simulink model "A2_TwoDOF_PID_task_space"  (R2014a)
settings: Solver=ode23t  StartTime=0.0  StopTime=10  FixedStep=1e-5  RelTol=1e-3
undefined symbols (not defined in the file): ADAMS_cwd, ADAMS_exec, ADAMS_host, ADAMS_init, ADAMS_inputs, ADAMS_outputs, ADAMS_prefix, ADAMS_static, ADAMS_sysdir
libraries: simulink x1
settings Model: Creator=Administrator  LastModifiedBy=Administrator
settings DebuggingCC: AlgebraicLoopMsg=none  SolverPrmCheckMsg=none

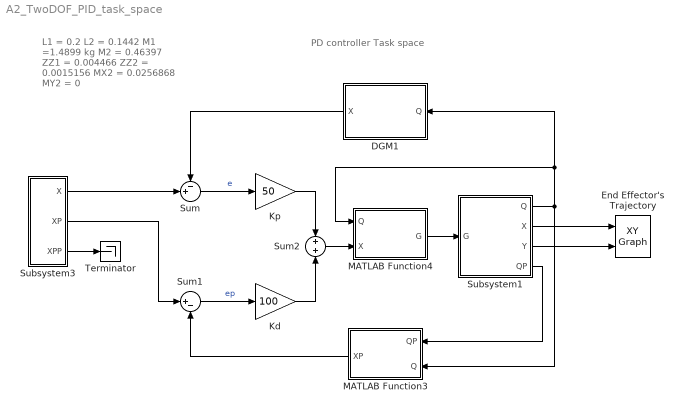
== system A2_TwoDOF_PID_task_space ==
  note: L1 = 0.2
      | L2 = 0.1442
      | M1 =1.4899 kg
      | M2 = 0.46397
      | ZZ1 = 0.004466
      | ZZ2 = 0.0015156
      | MX2 = 0.0256868
      | MY2 = 0
  note: PD controller Task space
  DGM1 : MATLAB Function  TreatAsAtomicUnit=on
  End Effector's Trajectory : simulink/Sinks/XY Graph  xmin=-0.5  xmax=0.5  ymin=-0.5  ymax=0.5  st=-1
  Kd : Gain  Gain=100
  Kp : Gain  Gain=50
  MATLAB Function3 : MATLAB Function  TreatAsAtomicUnit=on
  MATLAB Function4 : MATLAB Function  TreatAsAtomicUnit=on
  Subsystem1 : Subsystem
  Subsystem3 : Subsystem
  Sum : Sum  Inputs=-+|
  Sum1 : Sum  Inputs=|+-
  Sum2 : Sum  Inputs=+|+
  Terminator : Terminator
  wires:
  Subsystem1/1(Q) -> DGM1/1(Q), MATLAB Function4/1(Q), MATLAB Function3/2(Q)
  Subsystem1/2(X) -> End Effector's Trajectory/1
  Subsystem1/3(Y) -> End Effector's Trajectory/2
  Sum/1 -> Kp/1  "e"
  Sum1/1 -> Kd/1  "ep"
  Kp/1 -> Sum2/1
  Kd/1 -> Sum2/2
  DGM1/1(X) -> Sum/1
  Subsystem1/4(QP) -> MATLAB Function3/1(QP)
  MATLAB Function3/1(XP) -> Sum1/2
  Sum2/1 -> MATLAB Function4/2(X)
  MATLAB Function4/1(G) -> Subsystem1/1(G)
  Subsystem3/1(X) -> Sum/2
  Subsystem3/2(XP) -> Sum1/1
  Subsystem3/3(XPP) -> Terminator/1

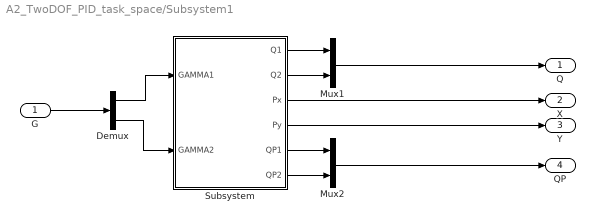
== system A2_TwoDOF_PID_task_space/Subsystem1 ==
  G : Inport
  Demux : Demux  Outputs=2
  Mux1 : Mux  Inputs=2
  Mux2 : Mux  Inputs=2
  Subsystem : Subsystem
  Q : Outport
  X : Outport  Port=2
  Y : Outport  Port=3
  QP : Outport  Port=4
  wires:
  Demux/2 -> Subsystem/2(GAMMA2)
  Subsystem/5(QP1) -> Mux2/1
  Subsystem/6(QP2) -> Mux2/2
  Demux/1 -> Subsystem/1(GAMMA1)
  Subsystem/4("Py ") -> Y/1
  Subsystem/3("Px ") -> X/1
  Subsystem/2("Q2 ") -> Mux1/2
  Mux1/1 -> Q/1
  Subsystem/1("Q1 ") -> Mux1/1
  Mux2/1 -> QP/1
  G/1 -> Demux/1

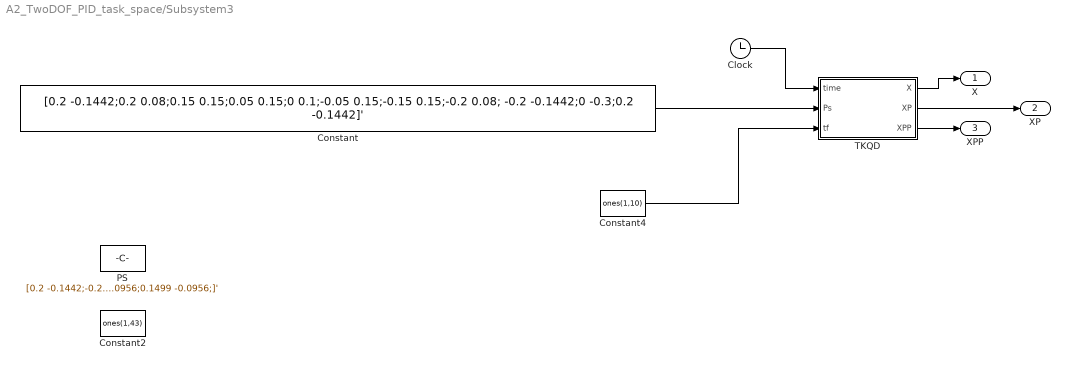
== system A2_TwoDOF_PID_task_space/Subsystem3 ==
  Clock : Clock
  Constant : Constant  Value=[0.2 -0.1442;0.2 0.08;0.15 0.15;0.05 0.15;0 0.1;-0.05 0.15;-0.15 0.15;-0.2 0.08; -0.2 -0.1442;0 -0.3;0.2 -0.1442]'
  Constant2 : Constant  Value=ones(1,43)
  Constant4 : Constant  Value=ones(1,10)
  PS : Constant  Value=[0.2 -0.1442;-0.2847 -0.0956;-0.2879 0.0916;-0.2673 0.0916;-0.2641 -0.0755;-0.1927 -0.0735;-0.1927 -0.0956;-0.2863 -0.0956;-0.1832 -0.0976;-0.1277 0.0936;-0.1087 0.0916;-0.0436 -0.0956;-0.0627 -0.0956;-0.0849 -0.0352;-0.1451 -0.0372;-0.1594 -0.0936;-0.1816 -0.0936;-0.0262 -0.0996;-0.0262 0.0936; 0.0040 0.0936; 0.0452 -0.0654; 0.0880 0.0916; 0.1134 0.0916; 0.1134 -0.0976; 0.0975 -0.0976; 0.0991 0.0574; 0.0531 -0.0956;0.0341 -0.0956;-0.0071 0.0614;-0.0087 -0.0956;-0.0262 -0.0956; 0.1499 -0.0956; 0.1499 0.0936; 0.2593 0.0936; 0.2578 0.0735; 0.1689 0.0735; 0.1689 0.0131; 0.2530 0.0131; 0.2530 -0.0070; 0.1705 -0.0070; 0.1721 -0.0775; 0.2625 -0.0775; 0.2625 -0.0956;0.1499 -0.0956;]'
  TKQD : MATLAB Function  TreatAsAtomicUnit=on
  X : Outport
  XP : Outport  Port=2
  XPP : Outport  Port=3
  wires:
  TKQD/2(XP) -> XP/1
  TKQD/3(XPP) -> XPP/1
  Clock/1 -> TKQD/1(time)
  TKQD/1(X) -> X/1
  Constant/1 -> TKQD/2(Ps)
  Constant4/1 -> TKQD/3(tf)

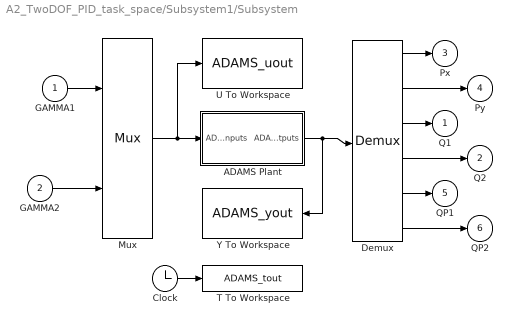
== system A2_TwoDOF_PID_task_space/Subsystem1/Subsystem ==
  GAMMA1 : Inport
  GAMMA2 : Inport  Port=2
  ADAMS Plant : Subsystem  LoadFcn=|  InitFcn=clear mex  mask(Adams Plant){exevie=ADAMS_sysdir, nam_in=ADAMS_inputs, namout=ADAMS_outputs, nampre=ADAMS_prefix, outfil=ADAMS_prefix, exesol=ADAMS_exec, stat=ADAMS_static, inicmd=[ADAMS_init], exetyp=C++, comtyp=PIPE(DDE), workdir=ADAMS_cwd, ada_host=ADAMS_host, modani=batch, modsim=continuous, dft=no, simulink_lead_cosim=yes, pin_interp_order=0, pout_extrap_order=0, pin_extrap_order=0, pout_interp_order=0, dt_out=0.005, o_rate=1, more=off}
      | %check based on dialog box setting for when setting by popup menu                                             
      | if exist('ADAMS_solver_type')                                                                                 
      |   if strcmp(ADAMS_solver_type,'C++')                                                                          
      |     set_param(gcb,'exetyp','C++');                                                                            
      |   else                                                                                                        
      |     set_param(gcb,'exetyp','Fortran');                                                                        
      |   end                                                                                                         
      | else                                                                                                          
      |   set_param(gcb,'exetyp','C++');                                                                              
      | end                                                                                                           
      | %set the mode if using acar_solver                                                                            
      | %REQUIRED HERE BECAUSE BELOW CAUSES MDLTERMINATE TO BE CALLED 2 TIMES IN MIDDLE OF SIMULATION WHEN SET IN MASK
      |                                                                                                               
      | %enable the direct feedthrough, sim mode, anim mode parameters by default                                     
      |                                                                                                               
      | if exist('set_some_params_states')                                                                            
      |                                                                                                               
      |   set_some_params_states({'dft','modsim','modani'},{'on','on','on'},'MaskEnables',gcb)                        
      |   %turn on direct feedthrough option                                                                          
      |   set_some_params_states({'dft'},{'on'},'MaskVisibilities',gcb)                                               
      |                                                                                                               
      |  end                                                                                                          
      |                                                                                                               
      |                                                                                                               
      | if exist('ADAMS_exec')                                                                                        
      |   if and(strcmp(get_param(gcb,'exesol'),'ADAMS_exec'),strcmp(ADAMS_exec,'acar_solver'))                       
      |     %set the sim mode to discrete -- only supported mode                                                      
      |     set_param(gcb,'modsim','discrete')                                                                        
      |      %turn off direct feedthrough option                                                                      
      |      set_some_params_states({'dft'},{'off'},'MaskVisibilities',gcb)                                           
      |     %set the animation mode to batch -- only supported mode                                                   
      |     set_param(gcb,'modani','batch')                                                                           
      |     %disable the direct feedthrough, sim mode, anim mode parameters                                           
      |     set_some_params_states({'modsim','modani'},{'off','off'},'MaskEnables',gcb)                               
      |   end                                                                                                         
      | end
      mask prompts: exevie "Adams install directory"; nam_in "Adams View input names"; namout "Adams View output names"; nampre "Adams model file prefix"; outfil "Output files prefix (opt.: if blank - no output)"; exesol "User executable (opt.: if blank - use standard)"; stat "Initial static simulation flag"; inicmd "Initialization commands"; exetyp "Adams Solver type"; comtyp "Interprocess option"; workdir "Adams working directory"; ada_host "Adams host"; modani "Animation mode"; modsim "Simulation mode"; dft "Direct feedthrough"; simulink_lead_cosim "Discrete Computational Order - Simulink Leads Adams"; pin_interp_order "Plant input interpolation order"; pout_extrap_order "Plant output extrapolation order"; pin_extrap_order "Plant input extrapolation order"; pout_interp_order "Plant output interpolation order"; dt_out "Communication interval"; o_rate "Number of communications per output step"; more "More parameters"
      mask help: Simulate any Adams plant model either in Adams Solver form (.adm file) or in Adams View form (.cmd file)
      settings: OpenFcn=|
      | open_system(gcb,'mask')
      | if not(exist('set_some_params_states'))
      | 
      | warning('The script "set_some_params_states.m" cannot be found in the MATLAB PATH.  Cannot update the ADAMS Plant S-Function parameters.')
      | 
      | warning('Recommended action(optional):  run the Adams Controls .m file first to help choose the correct settings in the Adams S-Function block.')
      | 
      | end
      mask Help:
      | <html>
      | This S-Function represents the non-linear Adams Plant with the inputs sent to the Adams model <br>
      |  and the outputs generated by the Adams model.  See the Adams Controls documentation for more <br>
      | information.  This plant uses the following variables:<br>
      | <br>
      | <b>ADAMS_sysdir  :</b> Adams installation directory<br>
      | <b>ADAMS_inputs  :</b> Input variables View names vector<br>
      | <b>ADAMS_outputs :</b> Outputs variables View names vector<br>
      | <b>ADAMS_prefix  : </b>ADAMS model files prefix (.adm, .cmd); also doubles as output files prefix<br>
      | <b>ADAMS_exec :</b> Adams Solver user library or keyword (e.g., acar_solver)<br>
      | <b>ADAMS_static :</b> yes|no - initial static before Co-simulation(discrete)/Function Evaluation(continuous)<br>
      | <b>ADAMS_init :</b>Initialization commands (i.e., Adams View or Solver commands, depending on setting for Animation mode)<br>
      | <b>ADAMS_cwd : </b> Current working directory (for TCP/IP)<br>
      | <b>ADAMS_host : </b>Name of Adams server host (for TCP/IP)<br>
      | <b>ADAMS_mode :</b> Linear or non-linear (i.e., co-sim, function eval)<br>
      | <b>ADAMS_solver_type :</b>Fortran or C++ (used to set popup menu when first loaded) <br>
      | 
      | 
      | <br>
      | The following settings can be chosen:<br>
      | <br>
      | <b>Adams Solver type:</b>  Fortran or C++ (will also set ADAMS_solver_type)<br>
      | <b>Interprocess option:</b> Pipe(DDE) or TCP/IP; TCP/IP can allow different machines run Adams and MATLAB<br>
      | <b>Animation mode:</b> batch (Solver, uses .adm) or interactive (View, uses .cmd)<br>
      | <b>Simulation mode:</b> discrete (Co-simulation) or continuous (Function Evaluation)<br>
      | <b>Discrete Computational Order - Simulink Lead Adams:</b> for discrete mode, chooses if Simulink leads the integration (yes) or lags (no);<br> if set to "no", can remove algebraic loop<br>
      | <b>Plant input interpolation order:</b> 0 = zero-order hold; 1 = linear (discrete mode only, where Simulink leads)<br>
      | <b>Plant output extrapolation order:</b> 0 = zero-order hold;1 = linear(discrete mode only, where Simulink leads)<br>
      | <b>Plant input extrapolation order:</b> 0 = zero-order hold; 1 = linear (discrete mode only, where Adams leads)<br>
      | <b>Plant output interpolation order:</b> 0 = zero-order hold;1 = linear(discrete mode only, where Adams leads)<br>
      | <b>Direct feedthrough:</b> yes|no - yes = Input directly effect output(continuous mode-only)<br>
      | <b>Communication interval:</b> Time step at which Co-simulation exchange information (e.g.,0.005); also controls <br>output for continuous mode (Function Evaluation)<br>
      | <b>Number of communications per output step: </b>Sets Adams output rate (.res, .req, .gra) integer value (default: 1)<br>
      | </html>
      mask Callback exesol:
      | if exist('set_some_params_states')
      | %enable the direct feedthrough, sim mode, anim mode parameters
      | set_some_params_states({'dft','modsim','modani'},{'on','on','on'},'MaskEnables',gcb)
      | %turn on direct feedthrough option
      | set_some_params_states({'dft'},{'on'},'MaskVisibilities',gcb)
      | end
      | 
      | if exist('ADAMS_exec')
      |   if and(strcmp(get_param(gcb,'exesol'),'ADAMS_exec'),strcmp(ADAMS_exec,'acar_solver'))
      |     %set the sim mode to discrete -- only supported mode
      |     %REMOVED:  BELOW CAUSES MDLTERMINATE TO BE CALLED 2 TIMES IN MIDDLE OF SIMULATION
      |     %Now in LoadFcn callback
      |     %set_param(gcb,'modsim','discrete')
      |      %turn off direct feedthrough option
      |     set_some_params_states({'dft'},{'off'},'MaskVisibilities',gcb)
      |     %set the animation mode to batch -- only supported mode
      |     %REMOVED:  BELOW CAUSES MDLTERMINATE TO BE CALLED 2 TIMES IN MIDDLE OF SIMULATION
      |     %Now in LoadFcn callback
      |     %set_param(gcb,'modani','batch')
      |     %disable the direct feedthrough, sim mode, anim mode parameters
      |     set_some_params_states({'modsim','modani'},{'off','off'},'MaskEnables',gcb)
      |   end
      | end
      mask TypeOptions exetyp: Fortran | C++
      mask Callback exetyp:
      | if strcmp(get_param(gcb,'exetyp'),'C++')
      |     ADAMS_solver_type='C++';
      | else
      |     ADAMS_solver_type='Fortran';
      | end
      mask TypeOptions comtyp: PIPE(DDE) | TCP/IP
      mask Callback comtyp:
      | if exist('set_some_params_states')
      | if strcmp(get_param(gcb,'comtyp'),'PIPE(DDE)')
      |     %turn off cwd, host options
      |     set_some_params_states({'ada_host','workdir'},{'off','off'},'MaskVisibilities',gcb)
      | else%if strcmp(get_param(gcb,'modsim'),'TCP/IP')
      |     %turn on cwd, host options
      |     set_some_params_states({'ada_host','workdir'},{'on','on'},'MaskVisibilities',gcb)
      | end
      | end
      mask TypeOptions modani: batch | interactive
      mask TypeOptions modsim: discrete | continuous
      mask Callback modsim:
      | if exist('set_some_params_states')
      | if strcmp(get_param(gcb,'modsim'),'discrete')
      |      %turn off direct feedthrough option
      |     set_some_params_states({'dft'},{'off'},'MaskVisibilities',gcb)
      |     %turn on discrete co-sim type if want to see more
      |     if strcmp(get_param(gcb,'more'),'on')
      |         set_some_params_states({'simulink_lead_cosim'},{'on'},'MaskVisibilities',gcb)
      |     end
      |     if strcmp(get_param(gcb,'simulink_lead_cosim'),'yes')
      |         %turn on interpolation/extrapolation options
      |         set_some_params_states({'pin_interp_order','pout_extrap_order',},{'on','on'},'MaskVisibilities',gcb)
      |     else
      |         set_some_params_states({'pin_extrap_order','pout_interp_order'},{'on','on'},'MaskVisibilities',gcb)
      |     end
      | else%if strcmp(get_param(gcb,'modsim'),'continuous')
      |      %turn off direct feedthrough option
      |     set_some_params_states({'dft'},{'on'},'MaskVisibilities',gcb)
      |     %turn off interpolation/extrapolation options
      |     set_some_params_states({'pin_interp_order','pout_extrap_order','pin_extrap_order','pout_interp_order','simulink_lead_cosim'},{'off','off','off','off','off'},'MaskVisibilities',gcb)
      | end
      | end
      mask TypeOptions dft: no | yes
      mask TypeOptions simulink_lead_cosim: yes | no
      mask Callback simulink_lead_cosim:
      | if exist('set_some_params_states')
      | if (strcmp(get_param(gcb,'simulink_lead_cosim'),'yes') && strcmp(get_param(gcb,'modsim'),'discrete'))
      |      %turn off unused interpolate/extrapolate options
      |     set_some_params_states({'pin_extrap_order','pout_interp_order'},{'off','off'},'MaskVisibilities',gcb)
      |     %turn on used interpolate/extrapolate options
      |     set_some_params_states({'pin_interp_order','pout_extrap_order'},{'on','on'},'MaskVisibilities',gcb)
      | elseif (strcmp(get_param(gcb,'simulink_lead_cosim'),'no') && strcmp(get_param(gcb,'modsim'),'discrete'))
      |     %turn on used interpolate/extrapolate options
      |     set_some_params_states({'pin_extrap_order','pout_interp_order'},{'on','on'},'MaskVisibilities',gcb)
      |      %turn off unused interpolate/extrapolate options
      |     set_some_params_states({'pin_interp_order','pout_extrap_order'},{'off','off'},'MaskVisibilities',gcb)
      | end
      | end
      mask TypeOptions pin_interp_order: 0 | 1
      mask TypeOptions pout_extrap_order: 0 | 1
      mask TypeOptions pin_extrap_order: 0 | 1
      mask TypeOptions pout_interp_order: 0 | 1
      mask Callback more:
      | if exist('set_some_params_states')
      | if (strcmp(get_param(gcb,'more'),'on'))
      |      %turn on infrequently used options
      |     set_some_params_states({'exevie','nam_in','namout','exesol','stat','inicmd'},{'on','on','on','on','on','on'},'MaskVisibilities',gcb)
      |     if strcmp(get_param(gcb,'modsim'),'discrete')
      |         set_some_params_states({'simulink_lead_cosim'},{'on'},'MaskVisibilities',gcb)
      |     end
      | elseif (strcmp(get_param(gcb,'more'),'off'))
      |     %turn off infrequently used options
      |     set_some_params_states({'exevie','nam_in','namout','exesol','stat','inicmd'},{'off','off','off','off','off','off'},'MaskVisibilities',gcb)
      |     if strcmp(get_param(gcb,'modsim'),'discrete')
      |         set_some_params_states({'simulink_lead_cosim'},{'off'},'MaskVisibilities',gcb)
      |     end
      | end
      | end
      mask Display: disp( 'MSC Software' )
  Clock : Clock
  Demux : Demux  Outputs=6
  Mux : Mux  Inputs=2
  T To Workspace : ToWorkspace  VariableName=ADAMS_tout
      settings: MaxDataPoints=100000
  U To Workspace : ToWorkspace  VariableName=ADAMS_uout
      settings: MaxDataPoints=100000
  Y To Workspace : ToWorkspace  VariableName=ADAMS_yout
      settings: MaxDataPoints=100000
  "Q1 " : Outport
  "Q2 " : Outport  Port=2
  "Px " : Outport  Port=3
  "Py " : Outport  Port=4
  QP1 : Outport  Port=5
  QP2 : Outport  Port=6
  wires:
  Clock/1 -> T To Workspace/1
  Mux/1 -> ADAMS Plant/1(ADAMS inputs), U To Workspace/1
  ADAMS Plant/1(ADAMS outputs) -> Demux/1, Y To Workspace/1
  Demux/1 -> "Px "/1
  Demux/2 -> "Py "/1
  Demux/3 -> "Q1 "/1
  Demux/4 -> "Q2 "/1
  Demux/5 -> QP1/1
  Demux/6 -> QP2/1
  GAMMA1/1 -> Mux/1
  GAMMA2/1 -> Mux/2

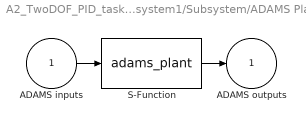
== system A2_TwoDOF_PID_task_space/Subsystem1/Subsystem/ADAMS Plant ==
  ADAMS inputs : Inport
  S-Function : S-Function  StopFcn=clear mex  FunctionName=adams_plant  Parameters=exevie,exesol,stat,outfil,nampre,o_rate,nam_in,namout,dft,modsim,modani,dt_out,inicmd,exetyp,comtyp,ada_host, workdir,pin_interp_order,pout_extrap_order,pin_extrap_order,pout_interp_order,simulink_lead_cosim  EnableBusSupport=off
  ADAMS outputs : Outport  InitialOutput=0
  wires:
  ADAMS inputs/1 -> S-Function/1
  S-Function/1 -> ADAMS outputs/1

== matlab function A2_TwoDOF_PID_task_space/Subsystem3/TKQD ==
  data: time input; X output; Ps input; tf input; XP output; XPP output
function [X,XP,XPP] = Quintic(time,Ps,tf)
% Calculate trajectory using Quintic polynomial
% r=10*(t/tf)^3-15*(t/tf)^4+6*(t/tf)^5;
% time is clock input
% Ps is the list of point = [P1 P2...]
% tf is the finish time for each interval
n=length(tf);
[k,tk_1] = find(time,tf,n);
if(k==1)
    t=min(time/tf(1),1);
else
    t = min((time-tk_1)/tf(k),1);
end
r=10*t^3-15*t^4+6*t^5;
rd=30*t^2-60*t^3+30*t^4;
r2d=60*t-180*t^2+120*t^3;
D=Ps(:,k+1)-Ps(:,k);
X=Ps(:,k)+r*D;
XP=rd*D;
XPP=r2d*D;
function [k,tk_1]=find(time,tf,n)
t=0;
k=n;
for i=1:n
    tk=t+tf(i);
    if(t<=time)&&(time<tk)
        k=i;
        break;
    end
    t=tk;
    if(i==n)
        t=tk-tf(n);
    end
end
tk_1=t;

== matlab function A2_TwoDOF_PID_task_space/MATLAB Function3 ==
  data: QP input; Q input; XP output
function XP  = JxQP(QP,Q)
%#codegen
C1 = cos(Q(1));
S1 = sin(Q(1));
C12 = cos(Q(1)+Q(2));
S12 = sin(Q(1)+Q(2));

L1 = 0.2;
L2 = 0.1442;

J1 = [-L1*S1-L2*S12, -L2*S12
      L1*C1+L2*C12, L2*C12];
XP = J1*QP;

== matlab function A2_TwoDOF_PID_task_space/MATLAB Function4 ==
  data: Q input; G output; X input
function G  = JT(Q,X)
%#codegen
C1 = cos(Q(1));
S1 = sin(Q(1));
C12 = cos(Q(1)+Q(2));
S12 = sin(Q(1)+Q(2));

L1 = 0.2;
L2 = 0.1442;

J = [-L1*S1-L2*S12, -L2*S12
      L1*C1+L2*C12, L2*C12];
G = J.'*X;

== matlab function A2_TwoDOF_PID_task_space/DGM1 ==
  data: Q input; X output
function X   = f(Q)
%#codegen
% Tested OK
L1 = 0.2;
L2 = 0.1442;
X1 = L1*cos(Q(1)) + L2*cos(Q(1)+Q(2));
X2 = L1*sin(Q(1)) + L2*sin(Q(1)+Q(2));
X = [X1;X2];
end
